simulink model "DriveSystemControl"  (R2025b)
settings: Solver=FixedStepAuto  StartTime=0.0  StopTime=Inf  FixedStep=0.001  RelTol=1e-3
PostLoadFcn:
  | if any(exist('dsrtsu_mdlpostloadfcn', 'file') ~= 0), dsrtsu_mdlpostloadfcn('Execute', bdroot); end
InitFcn:
  | , if any(exist('rtifpga_mdlclblib', 'file') ~= 0), rtifpga_mdlclblib('Init', bdroot); end,
  | , if any(exist('dsmpb_private', 'file') ~= 0), dsmpb_private('dsmpb_mdlclblib', 'Init', bdroot); end,
libraries: dsmpblib x2
(part 2 of 11)

== system DriveSystemControl/Bus Configuration (1) - In/Simulated ECUs/gitam Controller CAN File 08082024/BMS/TX/PDUs/BMS02 ==
  _BMS02_ : BusCreator  Inputs=4
  sigBatteryCurrent : Subsystem
  sigDriveCurrentLimit : Subsystem
  sigRegenCurrentLimit : Subsystem
  sigVehicleModeRequest : Subsystem
  BMS02 : Outport
  wires:
  _BMS02_/1 -> BMS02/1  "BMS02"
  sigVehicleModeRequest/1(sigVehicleModeRequest) -> _BMS02_/1  "sigVehicleModeRequest"
  sigRegenCurrentLimit/1(sigRegenCurrentLimit) -> _BMS02_/2  "sigRegenCurrentLimit"
  sigDriveCurrentLimit/1(sigDriveCurrentLimit) -> _BMS02_/3  "sigDriveCurrentLimit"
  sigBatteryCurrent/1(sigBatteryCurrent) -> _BMS02_/4  "sigBatteryCurrent"

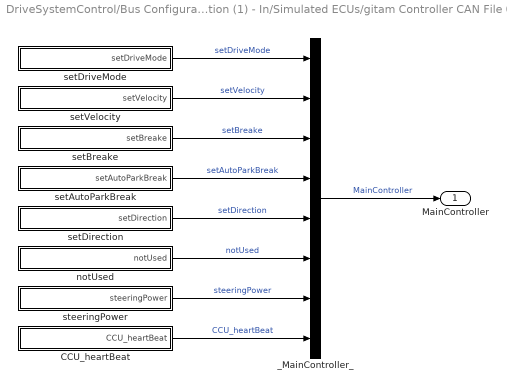
== system DriveSystemControl/Bus Configuration (1) - In/Simulated ECUs/gitam Controller CAN File 08082024/TCU/TX/PDUs/MainController ==
  CCU_heartBeat : Subsystem
  _MainController_ : BusCreator  Inputs=8
  notUsed : Subsystem
  setAutoParkBreak : Subsystem
  setBreake : Subsystem
  setDirection : Subsystem
  setDriveMode : Subsystem
  setVelocity : Subsystem
  steeringPower : Subsystem
  MainController : Outport
  wires:
  _MainController_/1 -> MainController/1  "MainController"
  setDriveMode/1(setDriveMode) -> _MainController_/1  "setDriveMode"
  setVelocity/1(setVelocity) -> _MainController_/2  "setVelocity"
  setBreake/1(setBreake) -> _MainController_/3  "setBreake"
  setAutoParkBreak/1(setAutoParkBreak) -> _MainController_/4  "setAutoParkBreak"
  setDirection/1(setDirection) -> _MainController_/5  "setDirection"
  notUsed/1(notUsed) -> _MainController_/6  "notUsed"
  steeringPower/1(steeringPower) -> _MainController_/7  "steeringPower"
  CCU_heartBeat/1(CCU_heartBeat) -> _MainController_/8  "CCU_heartBeat"

== system DriveSystemControl/Bus Configuration (1) - In/Simulated ECUs/gitam Controller CAN File 08082024/TCU/TX/PDUs/TCU01 ==
  _TCU01_ : BusCreator  Inputs=7
  sigBrake : Subsystem
  sigControllerTemperature : Subsystem
  sigDriveMode : Subsystem
  sigMotorTemperature : Subsystem
  sigRMSCurrent : Subsystem
  sigSpeed : Subsystem
  sigThrottle : Subsystem
  TCU01 : Outport
  wires:
  _TCU01_/1 -> TCU01/1  "TCU01"
  sigBrake/1(sigBrake) -> _TCU01_/1  "sigBrake"
  sigDriveMode/1(sigDriveMode) -> _TCU01_/2  "sigDriveMode"
  sigSpeed/1(sigSpeed) -> _TCU01_/3  "sigSpeed"
  sigThrottle/1(sigThrottle) -> _TCU01_/4  "sigThrottle"
  sigRMSCurrent/1(sigRMSCurrent) -> _TCU01_/5  "sigRMSCurrent"
  sigMotorTemperature/1(sigMotorTemperature) -> _TCU01_/6  "sigMotorTemperature"
  sigControllerTemperature/1(sigControllerTemperature) -> _TCU01_/7  "sigControllerTemperature"

== system DriveSystemControl/Bus Configuration (1) - In/Simulated ECUs/gitam Controller CAN File 08082024/TCU/TX/PDUs/TCU02 ==
  _TCU02_ : BusCreator  Inputs=3
  sigCapacitorVoltage : Subsystem
  sigMotorRPM : Subsystem
  sigOdometer : Subsystem
  TCU02 : Outport
  wires:
  _TCU02_/1 -> TCU02/1  "TCU02"
  sigOdometer/1(sigOdometer) -> _TCU02_/1  "sigOdometer"
  sigCapacitorVoltage/1(sigCapacitorVoltage) -> _TCU02_/2  "sigCapacitorVoltage"
  sigMotorRPM/1(sigMotorRPM) -> _TCU02_/3  "sigMotorRPM"

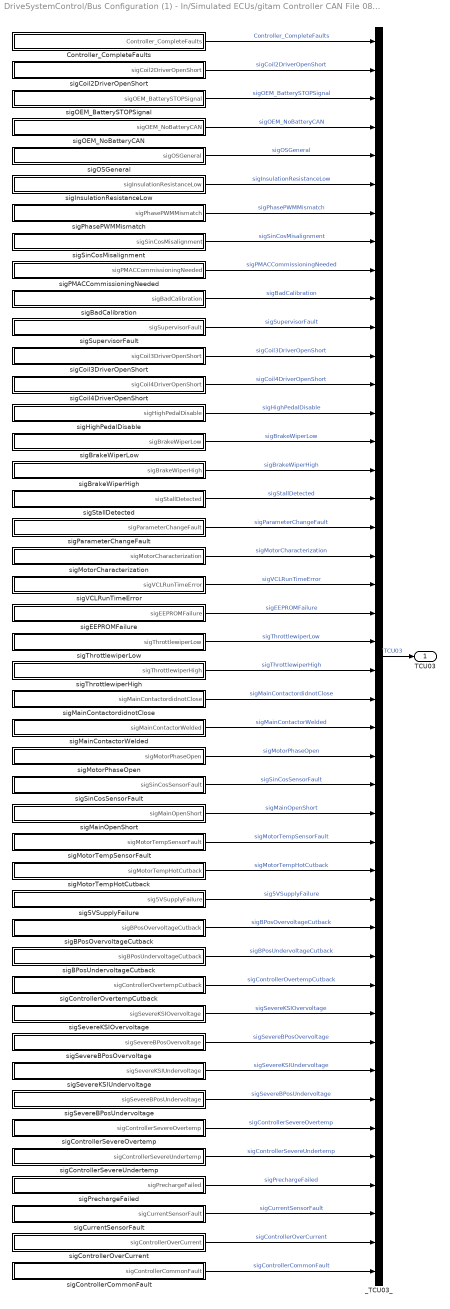
== system DriveSystemControl/Bus Configuration (1) - In/Simulated ECUs/gitam Controller CAN File 08082024/TCU/TX/PDUs/TCU03 ==
  Controller_CompleteFaults : Subsystem
  _TCU03_ : BusCreator  Inputs=44
  sig5VSupplyFailure : Subsystem
  sigBPosOvervoltageCutback : Subsystem
  sigBPosUndervoltageCutback : Subsystem
  sigBadCalibration : Subsystem
  sigBrakeWiperHigh : Subsystem
  sigBrakeWiperLow : Subsystem
  sigCoil2DriverOpenShort : Subsystem
  sigCoil3DriverOpenShort : Subsystem
  sigCoil4DriverOpenShort : Subsystem
  sigControllerCommonFault : Subsystem
  sigControllerOverCurrent : Subsystem
  sigControllerOvertempCutback : Subsystem
  sigControllerSevereOvertemp : Subsystem
  sigControllerSevereUndertemp : Subsystem
  sigCurrentSensorFault : Subsystem
  sigEEPROMFailure : Subsystem
  sigHighPedalDisable : Subsystem
  sigInsulationResistanceLow : Subsystem
  sigMainContactorWelded : Subsystem
  sigMainContactordidnotClose : Subsystem
  sigMainOpenShort : Subsystem
  sigMotorCharacterization : Subsystem
  sigMotorPhaseOpen : Subsystem
  sigMotorTempHotCutback : Subsystem
  sigMotorTempSensorFault : Subsystem
  sigOEM_BatterySTOPSignal : Subsystem
  sigOEM_NoBatteryCAN : Subsystem
  sigOSGeneral : Subsystem
  sigPMACCommissioningNeeded : Subsystem
  sigParameterChangeFault : Subsystem
  sigPhasePWMMismatch : Subsystem
  sigPrechargeFailed : Subsystem
  sigSevereBPosOvervoltage : Subsystem
  sigSevereBPosUndervoltage : Subsystem
  sigSevereKSIOvervoltage : Subsystem
  sigSevereKSIUndervoltage : Subsystem
  sigSinCosMisalignment : Subsystem
  sigSinCosSensorFault : Subsystem
  sigStallDetected : Subsystem
  sigSupervisorFault : Subsystem
  sigThrottlewiperHigh : Subsystem
  sigThrottlewiperLow : Subsystem
  sigVCLRunTimeError : Subsystem
  TCU03 : Outport
  wires:
  _TCU03_/1 -> TCU03/1  "TCU03"
  Controller_CompleteFaults/1(Controller_CompleteFaults) -> _TCU03_/1  "Controller_CompleteFaults"
  sigCoil2DriverOpenShort/1(sigCoil2DriverOpenShort) -> _TCU03_/2  "sigCoil2DriverOpenShort"
  sigOEM_BatterySTOPSignal/1(sigOEM_BatterySTOPSignal) -> _TCU03_/3  "sigOEM_BatterySTOPSignal"
  sigOEM_NoBatteryCAN/1(sigOEM_NoBatteryCAN) -> _TCU03_/4  "sigOEM_NoBatteryCAN"
  sigOSGeneral/1(sigOSGeneral) -> _TCU03_/5  "sigOSGeneral"
  sigInsulationResistanceLow/1(sigInsulationResistanceLow) -> _TCU03_/6  "sigInsulationResistanceLow"
  sigPhasePWMMismatch/1(sigPhasePWMMismatch) -> _TCU03_/7  "sigPhasePWMMismatch"
  sigSinCosMisalignment/1(sigSinCosMisalignment) -> _TCU03_/8  "sigSinCosMisalignment"
  sigPMACCommissioningNeeded/1(sigPMACCommissioningNeeded) -> _TCU03_/9  "sigPMACCommissioningNeeded"
  sigBadCalibration/1(sigBadCalibration) -> _TCU03_/10  "sigBadCalibration"
  sigSupervisorFault/1(sigSupervisorFault) -> _TCU03_/11  "sigSupervisorFault"
  sigCoil3DriverOpenShort/1(sigCoil3DriverOpenShort) -> _TCU03_/12  "sigCoil3DriverOpenShort"
  sigCoil4DriverOpenShort/1(sigCoil4DriverOpenShort) -> _TCU03_/13  "sigCoil4DriverOpenShort"
  sigHighPedalDisable/1(sigHighPedalDisable) -> _TCU03_/14  "sigHighPedalDisable"
  sigBrakeWiperLow/1(sigBrakeWiperLow) -> _TCU03_/15  "sigBrakeWiperLow"
  sigBrakeWiperHigh/1(sigBrakeWiperHigh) -> _TCU03_/16  "sigBrakeWiperHigh"
  sigStallDetected/1(sigStallDetected) -> _TCU03_/17  "sigStallDetected"
  sigParameterChangeFault/1(sigParameterChangeFault) -> _TCU03_/18  "sigParameterChangeFault"
  sigMotorCharacterization/1(sigMotorCharacterization) -> _TCU03_/19  "sigMotorCharacterization"
  sigVCLRunTimeError/1(sigVCLRunTimeError) -> _TCU03_/20  "sigVCLRunTimeError"
  sigEEPROMFailure/1(sigEEPROMFailure) -> _TCU03_/21  "sigEEPROMFailure"
  sigThrottlewiperLow/1(sigThrottlewiperLow) -> _TCU03_/22  "sigThrottlewiperLow"
  sigThrottlewiperHigh/1(sigThrottlewiperHigh) -> _TCU03_/23  "sigThrottlewiperHigh"
  sigMainContactordidnotClose/1(sigMainContactordidnotClose) -> _TCU03_/24  "sigMainContactordidnotClose"
  sigMainContactorWelded/1(sigMainContactorWelded) -> _TCU03_/25  "sigMainContactorWelded"
  sigMotorPhaseOpen/1(sigMotorPhaseOpen) -> _TCU03_/26  "sigMotorPhaseOpen"
  sigSinCosSensorFault/1(sigSinCosSensorFault) -> _TCU03_/27  "sigSinCosSensorFault"
  sigMainOpenShort/1(sigMainOpenShort) -> _TCU03_/28  "sigMainOpenShort"
  sigMotorTempSensorFault/1(sigMotorTempSensorFault) -> _TCU03_/29  "sigMotorTempSensorFault"
  sigMotorTempHotCutback/1(sigMotorTempHotCutback) -> _TCU03_/30  "sigMotorTempHotCutback"
  sig5VSupplyFailure/1(sig5VSupplyFailure) -> _TCU03_/31  "sig5VSupplyFailure"
  sigBPosOvervoltageCutback/1(sigBPosOvervoltageCutback) -> _TCU03_/32  "sigBPosOvervoltageCutback"
  sigBPosUndervoltageCutback/1(sigBPosUndervoltageCutback) -> _TCU03_/33  "sigBPosUndervoltageCutback"
  sigControllerOvertempCutback/1(sigControllerOvertempCutback) -> _TCU03_/34  "sigControllerOvertempCutback"
  sigSevereKSIOvervoltage/1(sigSevereKSIOvervoltage) -> _TCU03_/35  "sigSevereKSIOvervoltage"
  sigSevereBPosOvervoltage/1(sigSevereBPosOvervoltage) -> _TCU03_/36  "sigSevereBPosOvervoltage"
  sigSevereKSIUndervoltage/1(sigSevereKSIUndervoltage) -> _TCU03_/37  "sigSevereKSIUndervoltage"
  sigSevereBPosUndervoltage/1(sigSevereBPosUndervoltage) -> _TCU03_/38  "sigSevereBPosUndervoltage"
  sigControllerSevereOvertemp/1(sigControllerSevereOvertemp) -> _TCU03_/39  "sigControllerSevereOvertemp"
  sigControllerSevereUndertemp/1(sigControllerSevereUndertemp) -> _TCU03_/40  "sigControllerSevereUndertemp"
  sigPrechargeFailed/1(sigPrechargeFailed) -> _TCU03_/41  "sigPrechargeFailed"
  sigCurrentSensorFault/1(sigCurrentSensorFault) -> _TCU03_/42  "sigCurrentSensorFault"
  sigControllerOverCurrent/1(sigControllerOverCurrent) -> _TCU03_/43  "sigControllerOverCurrent"
  sigControllerCommonFault/1(sigControllerCommonFault) -> _TCU03_/44  "sigControllerCommonFault"

== system DriveSystemControl/Bus Configuration (1) - In/Simulated ECUs/gitam Controller CAN File 08082024/TCU/TX/PDUs/TCU04 ==
  _TCU04_ : BusCreator  Inputs=5
  sigMCU5_DriveMode : Subsystem
  sigMCU5_Efficiency : Subsystem
  sigMCU5_Hillhold : Subsystem
  sigMCU5_RegenFlag : Subsystem
  sigMCU5_Speed : Subsystem
  TCU04 : Outport
  wires:
  _TCU04_/1 -> TCU04/1  "TCU04"
  sigMCU5_Efficiency/1(sigMCU5_Efficiency) -> _TCU04_/1  "sigMCU5_Efficiency"
  sigMCU5_Hillhold/1(sigMCU5_Hillhold) -> _TCU04_/2  "sigMCU5_Hillhold"
  sigMCU5_Speed/1(sigMCU5_Speed) -> _TCU04_/3  "sigMCU5_Speed"
  sigMCU5_RegenFlag/1(sigMCU5_RegenFlag) -> _TCU04_/4  "sigMCU5_RegenFlag"
  sigMCU5_DriveMode/1(sigMCU5_DriveMode) -> _TCU04_/5  "sigMCU5_DriveMode"

== system DriveSystemControl/Bus Configuration (1) - In/Simulated ECUs/gitam Controller CAN File 08082024/TCU/TX/PDUs/TCU05 ==
  _TCU05_ : BusCreator  Inputs=1
  sigMCU6_Odometer : Subsystem
  TCU05 : Outport
  wires:
  _TCU05_/1 -> TCU05/1  "TCU05"
  sigMCU6_Odometer/1(sigMCU6_Odometer) -> _TCU05_/1  "sigMCU6_Odometer"

== system DriveSystemControl/Bus Configuration (1) - Out/Manipulation/gitam Controller CAN File 08082024/WIP/CANChannel/PDUs/BMS01 ==
  BMS01 : Inport
  _BMS01_ : BusSelector  OutputSignals=sigBatteryMalfunctionLight,sigKeyOnIndicator,sigStateOfCharge
  sigBatteryMalfunctionLight : Subsystem
  sigKeyOnIndicator : Subsystem
  sigStateOfCharge : Subsystem
  wires:
  BMS01/1 -> _BMS01_/1  "BMS01"
  _BMS01_/1 -> sigBatteryMalfunctionLight/1(sigBatteryMalfunctionLight)  "<sigBatteryMalfunctionLight>"
  _BMS01_/2 -> sigKeyOnIndicator/1(sigKeyOnIndicator)  "<sigKeyOnIndicator>"
  _BMS01_/3 -> sigStateOfCharge/1(sigStateOfCharge)  "<sigStateOfCharge>"

== system DriveSystemControl/Bus Configuration (1) - Out/Manipulation/gitam Controller CAN File 08082024/WIP/CANChannel/PDUs/BMS02 ==
  BMS02 : Inport
  _BMS02_ : BusSelector  OutputSignals=sigVehicleModeRequest,sigRegenCurrentLimit,sigDriveCurrentLimit,sigBatteryCurrent
  sigBatteryCurrent : Subsystem
  sigDriveCurrentLimit : Subsystem
  sigRegenCurrentLimit : Subsystem
  sigVehicleModeRequest : Subsystem
  wires:
  BMS02/1 -> _BMS02_/1  "BMS02"
  _BMS02_/1 -> sigVehicleModeRequest/1(sigVehicleModeRequest)  "<sigVehicleModeRequest>"
  _BMS02_/2 -> sigRegenCurrentLimit/1(sigRegenCurrentLimit)  "<sigRegenCurrentLimit>"
  _BMS02_/3 -> sigDriveCurrentLimit/1(sigDriveCurrentLimit)  "<sigDriveCurrentLimit>"
  _BMS02_/4 -> sigBatteryCurrent/1(sigBatteryCurrent)  "<sigBatteryCurrent>"

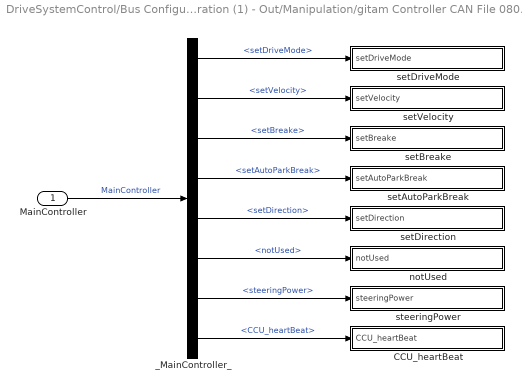
== system DriveSystemControl/Bus Configuration (1) - Out/Manipulation/gitam Controller CAN File 08082024/WIP/CANChannel/PDUs/MainController ==
  MainController : Inport
  CCU_heartBeat : Subsystem
  _MainController_ : BusSelector  OutputSignals=setDriveMode,setVelocity,setBreake,setAutoParkBreak,setDirection,notUsed,steeringPower,CCU_heartBeat
  notUsed : Subsystem
  setAutoParkBreak : Subsystem
  setBreake : Subsystem
  setDirection : Subsystem
  setDriveMode : Subsystem
  setVelocity : Subsystem
  steeringPower : Subsystem
  wires:
  MainController/1 -> _MainController_/1  "MainController"
  _MainController_/1 -> setDriveMode/1(setDriveMode)  "<setDriveMode>"
  _MainController_/2 -> setVelocity/1(setVelocity)  "<setVelocity>"
  _MainController_/3 -> setBreake/1(setBreake)  "<setBreake>"
  _MainController_/4 -> setAutoParkBreak/1(setAutoParkBreak)  "<setAutoParkBreak>"
  _MainController_/5 -> setDirection/1(setDirection)  "<setDirection>"
  _MainController_/6 -> notUsed/1(notUsed)  "<notUsed>"
  _MainController_/7 -> steeringPower/1(steeringPower)  "<steeringPower>"
  _MainController_/8 -> CCU_heartBeat/1(CCU_heartBeat)  "<CCU_heartBeat>"

== system DriveSystemControl/Bus Configuration (1) - Out/Manipulation/gitam Controller CAN File 08082024/WIP/CANChannel/PDUs/TCU01 ==
  TCU01 : Inport
  _TCU01_ : BusSelector  OutputSignals=sigBrake,sigDriveMode,sigSpeed,sigThrottle,sigRMSCurrent,sigMotorTemperature,sigControllerTemperature
  sigBrake : Subsystem
  sigControllerTemperature : Subsystem
  sigDriveMode : Subsystem
  sigMotorTemperature : Subsystem
  sigRMSCurrent : Subsystem
  sigSpeed : Subsystem
  sigThrottle : Subsystem
  wires:
  TCU01/1 -> _TCU01_/1  "TCU01"
  _TCU01_/1 -> sigBrake/1(sigBrake)  "<sigBrake>"
  _TCU01_/2 -> sigDriveMode/1(sigDriveMode)  "<sigDriveMode>"
  _TCU01_/3 -> sigSpeed/1(sigSpeed)  "<sigSpeed>"
  _TCU01_/4 -> sigThrottle/1(sigThrottle)  "<sigThrottle>"
  _TCU01_/5 -> sigRMSCurrent/1(sigRMSCurrent)  "<sigRMSCurrent>"
  _TCU01_/6 -> sigMotorTemperature/1(sigMotorTemperature)  "<sigMotorTemperature>"
  _TCU01_/7 -> sigControllerTemperature/1(sigControllerTemperature)  "<sigControllerTemperature>"

== system DriveSystemControl/Bus Configuration (1) - Out/Manipulation/gitam Controller CAN File 08082024/WIP/CANChannel/PDUs/TCU02 ==
  TCU02 : Inport
  _TCU02_ : BusSelector  OutputSignals=sigOdometer,sigCapacitorVoltage,sigMotorRPM
  sigCapacitorVoltage : Subsystem
  sigMotorRPM : Subsystem
  sigOdometer : Subsystem
  wires:
  TCU02/1 -> _TCU02_/1  "TCU02"
  _TCU02_/1 -> sigOdometer/1(sigOdometer)  "<sigOdometer>"
  _TCU02_/2 -> sigCapacitorVoltage/1(sigCapacitorVoltage)  "<sigCapacitorVoltage>"
  _TCU02_/3 -> sigMotorRPM/1(sigMotorRPM)  "<sigMotorRPM>"

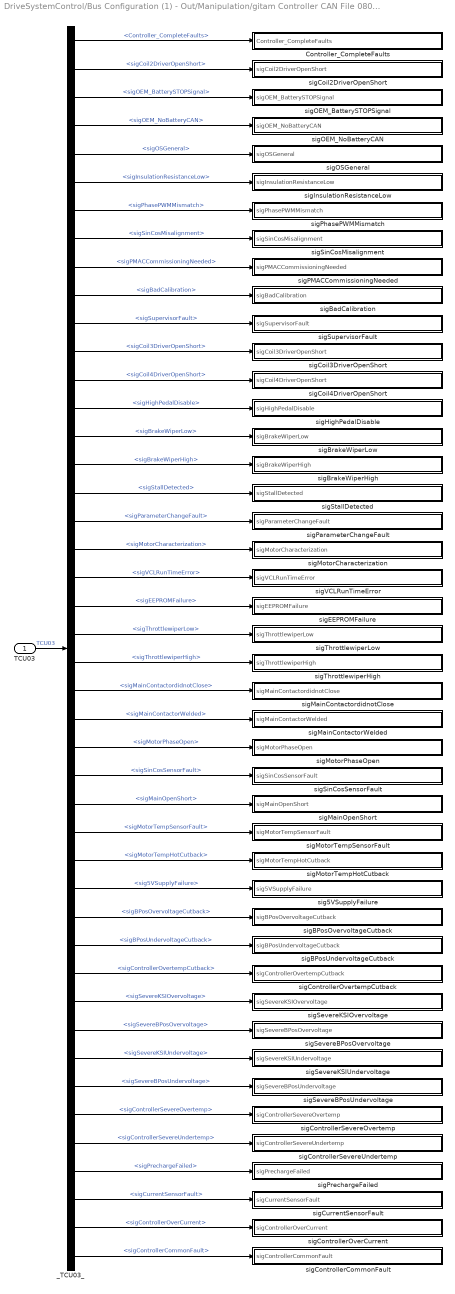
== system DriveSystemControl/Bus Configuration (1) - Out/Manipulation/gitam Controller CAN File 08082024/WIP/CANChannel/PDUs/TCU03 ==
  TCU03 : Inport
  Controller_CompleteFaults : Subsystem
  _TCU03_ : BusSelector  OutputSignals=Controller_CompleteFaults,sigCoil2DriverOpenShort,sigOEM_BatterySTOPSignal,sigOEM_NoBatteryCAN,sigOSGeneral,sigInsulationResistanceLow,sigPhasePWMMismatch,sigSinCosMisalignment,sigPMACCommissioningNeeded,sigBadCalibration,sigSupervisorFault,sigCoil3DriverOpenShort,sigCoil4DriverOpenShort,sigHighPedalDisable,sigBrakeWiperLow,sigBrakeWiperHigh,sigStallDetected,sigParameterChangeFault,sigMotorCharacterization,sigVCLRunTimeError,sigEEPROMFailure,sigThrottlewiperLow,sigThrottlewiperHigh,sigMainContactordidnotClose,sigMainContactorWelded,sigMotorPhaseOpen,sigSinCosSensorFault,sigMainOpenShort,sigMotorTempSensorFault,sigMotorTempHotCutback,sig5VSupplyFailure,sigBPosOvervoltageCutback,sigBPosUndervoltageCutback,sigControllerOvertempCutback,sigSevereKSIOvervoltage,sigSevereBPosOvervoltage,sigSevereKSIUndervoltage,sigSevereBPosUndervoltage,sigControllerSevereOvertemp,sigControllerSevereUndertemp,sigPrechargeFailed,sigCurrentSensorFault,sigControllerOverCurrent,sigControllerCommonFault
  sig5VSupplyFailure : Subsystem
  sigBPosOvervoltageCutback : Subsystem
  sigBPosUndervoltageCutback : Subsystem
  sigBadCalibration : Subsystem
  sigBrakeWiperHigh : Subsystem
  sigBrakeWiperLow : Subsystem
  sigCoil2DriverOpenShort : Subsystem
  sigCoil3DriverOpenShort : Subsystem
  sigCoil4DriverOpenShort : Subsystem
  sigControllerCommonFault : Subsystem
  sigControllerOverCurrent : Subsystem
  sigControllerOvertempCutback : Subsystem
  sigControllerSevereOvertemp : Subsystem
  sigControllerSevereUndertemp : Subsystem
  sigCurrentSensorFault : Subsystem
  sigEEPROMFailure : Subsystem
  sigHighPedalDisable : Subsystem
  sigInsulationResistanceLow : Subsystem
  sigMainContactorWelded : Subsystem
  sigMainContactordidnotClose : Subsystem
  sigMainOpenShort : Subsystem
  sigMotorCharacterization : Subsystem
  sigMotorPhaseOpen : Subsystem
  sigMotorTempHotCutback : Subsystem
  sigMotorTempSensorFault : Subsystem
  sigOEM_BatterySTOPSignal : Subsystem
  sigOEM_NoBatteryCAN : Subsystem
  sigOSGeneral : Subsystem
  sigPMACCommissioningNeeded : Subsystem
  sigParameterChangeFault : Subsystem
  sigPhasePWMMismatch : Subsystem
  sigPrechargeFailed : Subsystem
  sigSevereBPosOvervoltage : Subsystem
  sigSevereBPosUndervoltage : Subsystem
  sigSevereKSIOvervoltage : Subsystem
  sigSevereKSIUndervoltage : Subsystem
  sigSinCosMisalignment : Subsystem
  sigSinCosSensorFault : Subsystem
  sigStallDetected : Subsystem
  sigSupervisorFault : Subsystem
  sigThrottlewiperHigh : Subsystem
  sigThrottlewiperLow : Subsystem
  sigVCLRunTimeError : Subsystem
  wires:
  TCU03/1 -> _TCU03_/1  "TCU03"
  _TCU03_/1 -> Controller_CompleteFaults/1(Controller_CompleteFaults)  "<Controller_CompleteFaults>"
  _TCU03_/2 -> sigCoil2DriverOpenShort/1(sigCoil2DriverOpenShort)  "<sigCoil2DriverOpenShort>"
  _TCU03_/3 -> sigOEM_BatterySTOPSignal/1(sigOEM_BatterySTOPSignal)  "<sigOEM_BatterySTOPSignal>"
  _TCU03_/4 -> sigOEM_NoBatteryCAN/1(sigOEM_NoBatteryCAN)  "<sigOEM_NoBatteryCAN>"
  _TCU03_/5 -> sigOSGeneral/1(sigOSGeneral)  "<sigOSGeneral>"
  _TCU03_/6 -> sigInsulationResistanceLow/1(sigInsulationResistanceLow)  "<sigInsulationResistanceLow>"
  _TCU03_/7 -> sigPhasePWMMismatch/1(sigPhasePWMMismatch)  "<sigPhasePWMMismatch>"
  _TCU03_/8 -> sigSinCosMisalignment/1(sigSinCosMisalignment)  "<sigSinCosMisalignment>"
  _TCU03_/9 -> sigPMACCommissioningNeeded/1(sigPMACCommissioningNeeded)  "<sigPMACCommissioningNeeded>"
  _TCU03_/10 -> sigBadCalibration/1(sigBadCalibration)  "<sigBadCalibration>"
  _TCU03_/11 -> sigSupervisorFault/1(sigSupervisorFault)  "<sigSupervisorFault>"
  _TCU03_/12 -> sigCoil3DriverOpenShort/1(sigCoil3DriverOpenShort)  "<sigCoil3DriverOpenShort>"
  _TCU03_/13 -> sigCoil4DriverOpenShort/1(sigCoil4DriverOpenShort)  "<sigCoil4DriverOpenShort>"
  _TCU03_/14 -> sigHighPedalDisable/1(sigHighPedalDisable)  "<sigHighPedalDisable>"
  _TCU03_/15 -> sigBrakeWiperLow/1(sigBrakeWiperLow)  "<sigBrakeWiperLow>"
  _TCU03_/16 -> sigBrakeWiperHigh/1(sigBrakeWiperHigh)  "<sigBrakeWiperHigh>"
  _TCU03_/17 -> sigStallDetected/1(sigStallDetected)  "<sigStallDetected>"
  _TCU03_/18 -> sigParameterChangeFault/1(sigParameterChangeFault)  "<sigParameterChangeFault>"
  _TCU03_/19 -> sigMotorCharacterization/1(sigMotorCharacterization)  "<sigMotorCharacterization>"
  _TCU03_/20 -> sigVCLRunTimeError/1(sigVCLRunTimeError)  "<sigVCLRunTimeError>"
  _TCU03_/21 -> sigEEPROMFailure/1(sigEEPROMFailure)  "<sigEEPROMFailure>"
  _TCU03_/22 -> sigThrottlewiperLow/1(sigThrottlewiperLow)  "<sigThrottlewiperLow>"
  _TCU03_/23 -> sigThrottlewiperHigh/1(sigThrottlewiperHigh)  "<sigThrottlewiperHigh>"
  _TCU03_/24 -> sigMainContactordidnotClose/1(sigMainContactordidnotClose)  "<sigMainContactordidnotClose>"
  _TCU03_/25 -> sigMainContactorWelded/1(sigMainContactorWelded)  "<sigMainContactorWelded>"
  _TCU03_/26 -> sigMotorPhaseOpen/1(sigMotorPhaseOpen)  "<sigMotorPhaseOpen>"
  _TCU03_/27 -> sigSinCosSensorFault/1(sigSinCosSensorFault)  "<sigSinCosSensorFault>"
  _TCU03_/28 -> sigMainOpenShort/1(sigMainOpenShort)  "<sigMainOpenShort>"
  _TCU03_/29 -> sigMotorTempSensorFault/1(sigMotorTempSensorFault)  "<sigMotorTempSensorFault>"
  _TCU03_/30 -> sigMotorTempHotCutback/1(sigMotorTempHotCutback)  "<sigMotorTempHotCutback>"
  _TCU03_/31 -> sig5VSupplyFailure/1(sig5VSupplyFailure)  "<sig5VSupplyFailure>"
  _TCU03_/32 -> sigBPosOvervoltageCutback/1(sigBPosOvervoltageCutback)  "<sigBPosOvervoltageCutback>"
  _TCU03_/33 -> sigBPosUndervoltageCutback/1(sigBPosUndervoltageCutback)  "<sigBPosUndervoltageCutback>"
  _TCU03_/34 -> sigControllerOvertempCutback/1(sigControllerOvertempCutback)  "<sigControllerOvertempCutback>"
  _TCU03_/35 -> sigSevereKSIOvervoltage/1(sigSevereKSIOvervoltage)  "<sigSevereKSIOvervoltage>"
  _TCU03_/36 -> sigSevereBPosOvervoltage/1(sigSevereBPosOvervoltage)  "<sigSevereBPosOvervoltage>"
  _TCU03_/37 -> sigSevereKSIUndervoltage/1(sigSevereKSIUndervoltage)  "<sigSevereKSIUndervoltage>"
  _TCU03_/38 -> sigSevereBPosUndervoltage/1(sigSevereBPosUndervoltage)  "<sigSevereBPosUndervoltage>"
  _TCU03_/39 -> sigControllerSevereOvertemp/1(sigControllerSevereOvertemp)  "<sigControllerSevereOvertemp>"
  _TCU03_/40 -> sigControllerSevereUndertemp/1(sigControllerSevereUndertemp)  "<sigControllerSevereUndertemp>"
  _TCU03_/41 -> sigPrechargeFailed/1(sigPrechargeFailed)  "<sigPrechargeFailed>"
  _TCU03_/42 -> sigCurrentSensorFault/1(sigCurrentSensorFault)  "<sigCurrentSensorFault>"
  _TCU03_/43 -> sigControllerOverCurrent/1(sigControllerOverCurrent)  "<sigControllerOverCurrent>"
  _TCU03_/44 -> sigControllerCommonFault/1(sigControllerCommonFault)  "<sigControllerCommonFault>"

== system DriveSystemControl/Bus Configuration (1) - Out/Manipulation/gitam Controller CAN File 08082024/WIP/CANChannel/PDUs/TCU04 ==
  TCU04 : Inport
  _TCU04_ : BusSelector  OutputSignals=sigMCU5_Efficiency,sigMCU5_Hillhold,sigMCU5_Speed,sigMCU5_RegenFlag,sigMCU5_DriveMode
  sigMCU5_DriveMode : Subsystem
  sigMCU5_Efficiency : Subsystem
  sigMCU5_Hillhold : Subsystem
  sigMCU5_RegenFlag : Subsystem
  sigMCU5_Speed : Subsystem
  wires:
  TCU04/1 -> _TCU04_/1  "TCU04"
  _TCU04_/1 -> sigMCU5_Efficiency/1(sigMCU5_Efficiency)  "<sigMCU5_Efficiency>"
  _TCU04_/2 -> sigMCU5_Hillhold/1(sigMCU5_Hillhold)  "<sigMCU5_Hillhold>"
  _TCU04_/3 -> sigMCU5_Speed/1(sigMCU5_Speed)  "<sigMCU5_Speed>"
  _TCU04_/4 -> sigMCU5_RegenFlag/1(sigMCU5_RegenFlag)  "<sigMCU5_RegenFlag>"
  _TCU04_/5 -> sigMCU5_DriveMode/1(sigMCU5_DriveMode)  "<sigMCU5_DriveMode>"

== system DriveSystemControl/Bus Configuration (1) - Out/Manipulation/gitam Controller CAN File 08082024/WIP/CANChannel/PDUs/TCU05 ==
  TCU05 : Inport
  _TCU05_ : BusSelector  OutputSignals=sigMCU6_Odometer
  sigMCU6_Odometer : Subsystem
  wires:
  TCU05/1 -> _TCU05_/1  "TCU05"
  _TCU05_/1 -> sigMCU6_Odometer/1(sigMCU6_Odometer)  "<sigMCU6_Odometer>"

== system DriveSystemControl/Bus Configuration (1) - Out/Simulated ECUs/gitam Controller CAN File 08082024/BMS/RX/PDUs/TCU04 ==
  TCU04 : Inport
  _TCU04_ : BusSelector  OutputSignals=sigMCU5_Efficiency,sigMCU5_Hillhold,sigMCU5_Speed,sigMCU5_RegenFlag,sigMCU5_DriveMode
  sigMCU5_DriveMode : Subsystem
  sigMCU5_Efficiency : Subsystem
  sigMCU5_Hillhold : Subsystem
  sigMCU5_RegenFlag : Subsystem
  sigMCU5_Speed : Subsystem
  wires:
  TCU04/1 -> _TCU04_/1  "TCU04"
  _TCU04_/1 -> sigMCU5_Efficiency/1(sigMCU5_Efficiency)  "<sigMCU5_Efficiency>"
  _TCU04_/2 -> sigMCU5_Hillhold/1(sigMCU5_Hillhold)  "<sigMCU5_Hillhold>"
  _TCU04_/3 -> sigMCU5_Speed/1(sigMCU5_Speed)  "<sigMCU5_Speed>"
  _TCU04_/4 -> sigMCU5_RegenFlag/1(sigMCU5_RegenFlag)  "<sigMCU5_RegenFlag>"
  _TCU04_/5 -> sigMCU5_DriveMode/1(sigMCU5_DriveMode)  "<sigMCU5_DriveMode>"

== system DriveSystemControl/Bus Configuration (1) - Out/Simulated ECUs/gitam Controller CAN File 08082024/IPC/RX/PDUs/BMS01 ==
  BMS01 : Inport
  _BMS01_ : BusSelector  OutputSignals=sigBatteryMalfunctionLight,sigKeyOnIndicator,sigStateOfCharge
  sigBatteryMalfunctionLight : Subsystem
  sigKeyOnIndicator : Subsystem
  sigStateOfCharge : Subsystem
  wires:
  BMS01/1 -> _BMS01_/1  "BMS01"
  _BMS01_/1 -> sigBatteryMalfunctionLight/1(sigBatteryMalfunctionLight)  "<sigBatteryMalfunctionLight>"
  _BMS01_/2 -> sigKeyOnIndicator/1(sigKeyOnIndicator)  "<sigKeyOnIndicator>"
  _BMS01_/3 -> sigStateOfCharge/1(sigStateOfCharge)  "<sigStateOfCharge>"

== system DriveSystemControl/Bus Configuration (1) - Out/Simulated ECUs/gitam Controller CAN File 08082024/IPC/RX/PDUs/TCU01 ==
  TCU01 : Inport
  _TCU01_ : BusSelector  OutputSignals=sigBrake,sigDriveMode,sigSpeed,sigThrottle,sigRMSCurrent,sigMotorTemperature,sigControllerTemperature
  sigBrake : Subsystem
  sigControllerTemperature : Subsystem
  sigDriveMode : Subsystem
  sigMotorTemperature : Subsystem
  sigRMSCurrent : Subsystem
  sigSpeed : Subsystem
  sigThrottle : Subsystem
  wires:
  TCU01/1 -> _TCU01_/1  "TCU01"
  _TCU01_/1 -> sigBrake/1(sigBrake)  "<sigBrake>"
  _TCU01_/2 -> sigDriveMode/1(sigDriveMode)  "<sigDriveMode>"
  _TCU01_/3 -> sigSpeed/1(sigSpeed)  "<sigSpeed>"
  _TCU01_/4 -> sigThrottle/1(sigThrottle)  "<sigThrottle>"
  _TCU01_/5 -> sigRMSCurrent/1(sigRMSCurrent)  "<sigRMSCurrent>"
  _TCU01_/6 -> sigMotorTemperature/1(sigMotorTemperature)  "<sigMotorTemperature>"
  _TCU01_/7 -> sigControllerTemperature/1(sigControllerTemperature)  "<sigControllerTemperature>"

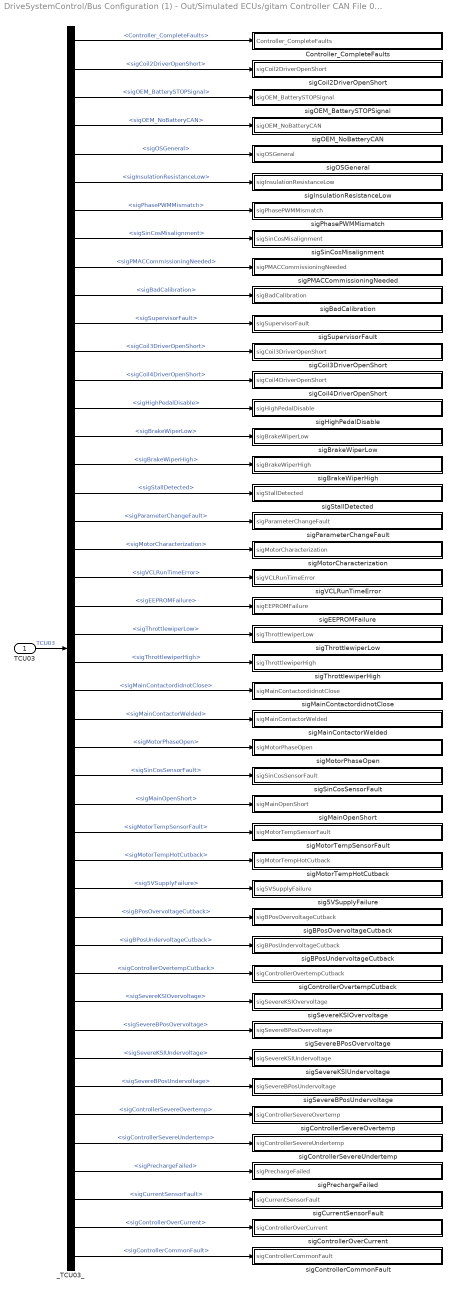
== system DriveSystemControl/Bus Configuration (1) - Out/Simulated ECUs/gitam Controller CAN File 08082024/IPC/RX/PDUs/TCU03 ==
  TCU03 : Inport
  Controller_CompleteFaults : Subsystem
  _TCU03_ : BusSelector  OutputSignals=Controller_CompleteFaults,sigCoil2DriverOpenShort,sigOEM_BatterySTOPSignal,sigOEM_NoBatteryCAN,sigOSGeneral,sigInsulationResistanceLow,sigPhasePWMMismatch,sigSinCosMisalignment,sigPMACCommissioningNeeded,sigBadCalibration,sigSupervisorFault,sigCoil3DriverOpenShort,sigCoil4DriverOpenShort,sigHighPedalDisable,sigBrakeWiperLow,sigBrakeWiperHigh,sigStallDetected,sigParameterChangeFault,sigMotorCharacterization,sigVCLRunTimeError,sigEEPROMFailure,sigThrottlewiperLow,sigThrottlewiperHigh,sigMainContactordidnotClose,sigMainContactorWelded,sigMotorPhaseOpen,sigSinCosSensorFault,sigMainOpenShort,sigMotorTempSensorFault,sigMotorTempHotCutback,sig5VSupplyFailure,sigBPosOvervoltageCutback,sigBPosUndervoltageCutback,sigControllerOvertempCutback,sigSevereKSIOvervoltage,sigSevereBPosOvervoltage,sigSevereKSIUndervoltage,sigSevereBPosUndervoltage,sigControllerSevereOvertemp,sigControllerSevereUndertemp,sigPrechargeFailed,sigCurrentSensorFault,sigControllerOverCurrent,sigControllerCommonFault
  sig5VSupplyFailure : Subsystem
  sigBPosOvervoltageCutback : Subsystem
  sigBPosUndervoltageCutback : Subsystem
  sigBadCalibration : Subsystem
  sigBrakeWiperHigh : Subsystem
  sigBrakeWiperLow : Subsystem
  sigCoil2DriverOpenShort : Subsystem
  sigCoil3DriverOpenShort : Subsystem
  sigCoil4DriverOpenShort : Subsystem
  sigControllerCommonFault : Subsystem
  sigControllerOverCurrent : Subsystem
  sigControllerOvertempCutback : Subsystem
  sigControllerSevereOvertemp : Subsystem
  sigControllerSevereUndertemp : Subsystem
  sigCurrentSensorFault : Subsystem
  sigEEPROMFailure : Subsystem
  sigHighPedalDisable : Subsystem
  sigInsulationResistanceLow : Subsystem
  sigMainContactorWelded : Subsystem
  sigMainContactordidnotClose : Subsystem
  sigMainOpenShort : Subsystem
  sigMotorCharacterization : Subsystem
  sigMotorPhaseOpen : Subsystem
  sigMotorTempHotCutback : Subsystem
  sigMotorTempSensorFault : Subsystem
  sigOEM_BatterySTOPSignal : Subsystem
  sigOEM_NoBatteryCAN : Subsystem
  sigOSGeneral : Subsystem
  sigPMACCommissioningNeeded : Subsystem
  sigParameterChangeFault : Subsystem
  sigPhasePWMMismatch : Subsystem
  sigPrechargeFailed : Subsystem
  sigSevereBPosOvervoltage : Subsystem
  sigSevereBPosUndervoltage : Subsystem
  sigSevereKSIOvervoltage : Subsystem
  sigSevereKSIUndervoltage : Subsystem
  sigSinCosMisalignment : Subsystem
  sigSinCosSensorFault : Subsystem
  sigStallDetected : Subsystem
  sigSupervisorFault : Subsystem
  sigThrottlewiperHigh : Subsystem
  sigThrottlewiperLow : Subsystem
  sigVCLRunTimeError : Subsystem
  wires:
  TCU03/1 -> _TCU03_/1  "TCU03"
  _TCU03_/1 -> Controller_CompleteFaults/1(Controller_CompleteFaults)  "<Controller_CompleteFaults>"
  _TCU03_/2 -> sigCoil2DriverOpenShort/1(sigCoil2DriverOpenShort)  "<sigCoil2DriverOpenShort>"
  _TCU03_/3 -> sigOEM_BatterySTOPSignal/1(sigOEM_BatterySTOPSignal)  "<sigOEM_BatterySTOPSignal>"
  _TCU03_/4 -> sigOEM_NoBatteryCAN/1(sigOEM_NoBatteryCAN)  "<sigOEM_NoBatteryCAN>"
  _TCU03_/5 -> sigOSGeneral/1(sigOSGeneral)  "<sigOSGeneral>"
  _TCU03_/6 -> sigInsulationResistanceLow/1(sigInsulationResistanceLow)  "<sigInsulationResistanceLow>"
  _TCU03_/7 -> sigPhasePWMMismatch/1(sigPhasePWMMismatch)  "<sigPhasePWMMismatch>"
  _TCU03_/8 -> sigSinCosMisalignment/1(sigSinCosMisalignment)  "<sigSinCosMisalignment>"
  _TCU03_/9 -> sigPMACCommissioningNeeded/1(sigPMACCommissioningNeeded)  "<sigPMACCommissioningNeeded>"
  _TCU03_/10 -> sigBadCalibration/1(sigBadCalibration)  "<sigBadCalibration>"
  _TCU03_/11 -> sigSupervisorFault/1(sigSupervisorFault)  "<sigSupervisorFault>"
  _TCU03_/12 -> sigCoil3DriverOpenShort/1(sigCoil3DriverOpenShort)  "<sigCoil3DriverOpenShort>"
  _TCU03_/13 -> sigCoil4DriverOpenShort/1(sigCoil4DriverOpenShort)  "<sigCoil4DriverOpenShort>"
  _TCU03_/14 -> sigHighPedalDisable/1(sigHighPedalDisable)  "<sigHighPedalDisable>"
  _TCU03_/15 -> sigBrakeWiperLow/1(sigBrakeWiperLow)  "<sigBrakeWiperLow>"
  _TCU03_/16 -> sigBrakeWiperHigh/1(sigBrakeWiperHigh)  "<sigBrakeWiperHigh>"
  _TCU03_/17 -> sigStallDetected/1(sigStallDetected)  "<sigStallDetected>"
  _TCU03_/18 -> sigParameterChangeFault/1(sigParameterChangeFault)  "<sigParameterChangeFault>"
  _TCU03_/19 -> sigMotorCharacterization/1(sigMotorCharacterization)  "<sigMotorCharacterization>"
  _TCU03_/20 -> sigVCLRunTimeError/1(sigVCLRunTimeError)  "<sigVCLRunTimeError>"
  _TCU03_/21 -> sigEEPROMFailure/1(sigEEPROMFailure)  "<sigEEPROMFailure>"
  _TCU03_/22 -> sigThrottlewiperLow/1(sigThrottlewiperLow)  "<sigThrottlewiperLow>"
  _TCU03_/23 -> sigThrottlewiperHigh/1(sigThrottlewiperHigh)  "<sigThrottlewiperHigh>"
  _TCU03_/24 -> sigMainContactordidnotClose/1(sigMainContactordidnotClose)  "<sigMainContactordidnotClose>"
  _TCU03_/25 -> sigMainContactorWelded/1(sigMainContactorWelded)  "<sigMainContactorWelded>"
  _TCU03_/26 -> sigMotorPhaseOpen/1(sigMotorPhaseOpen)  "<sigMotorPhaseOpen>"
  _TCU03_/27 -> sigSinCosSensorFault/1(sigSinCosSensorFault)  "<sigSinCosSensorFault>"
  _TCU03_/28 -> sigMainOpenShort/1(sigMainOpenShort)  "<sigMainOpenShort>"
  _TCU03_/29 -> sigMotorTempSensorFault/1(sigMotorTempSensorFault)  "<sigMotorTempSensorFault>"
  _TCU03_/30 -> sigMotorTempHotCutback/1(sigMotorTempHotCutback)  "<sigMotorTempHotCutback>"
  _TCU03_/31 -> sig5VSupplyFailure/1(sig5VSupplyFailure)  "<sig5VSupplyFailure>"
  _TCU03_/32 -> sigBPosOvervoltageCutback/1(sigBPosOvervoltageCutback)  "<sigBPosOvervoltageCutback>"
  _TCU03_/33 -> sigBPosUndervoltageCutback/1(sigBPosUndervoltageCutback)  "<sigBPosUndervoltageCutback>"
  _TCU03_/34 -> sigControllerOvertempCutback/1(sigControllerOvertempCutback)  "<sigControllerOvertempCutback>"
  _TCU03_/35 -> sigSevereKSIOvervoltage/1(sigSevereKSIOvervoltage)  "<sigSevereKSIOvervoltage>"
  _TCU03_/36 -> sigSevereBPosOvervoltage/1(sigSevereBPosOvervoltage)  "<sigSevereBPosOvervoltage>"
  _TCU03_/37 -> sigSevereKSIUndervoltage/1(sigSevereKSIUndervoltage)  "<sigSevereKSIUndervoltage>"
  _TCU03_/38 -> sigSevereBPosUndervoltage/1(sigSevereBPosUndervoltage)  "<sigSevereBPosUndervoltage>"
  _TCU03_/39 -> sigControllerSevereOvertemp/1(sigControllerSevereOvertemp)  "<sigControllerSevereOvertemp>"
  _TCU03_/40 -> sigControllerSevereUndertemp/1(sigControllerSevereUndertemp)  "<sigControllerSevereUndertemp>"
  _TCU03_/41 -> sigPrechargeFailed/1(sigPrechargeFailed)  "<sigPrechargeFailed>"
  _TCU03_/42 -> sigCurrentSensorFault/1(sigCurrentSensorFault)  "<sigCurrentSensorFault>"
  _TCU03_/43 -> sigControllerOverCurrent/1(sigControllerOverCurrent)  "<sigControllerOverCurrent>"
  _TCU03_/44 -> sigControllerCommonFault/1(sigControllerCommonFault)  "<sigControllerCommonFault>"

== system DriveSystemControl/Bus Configuration (1) - Out/Simulated ECUs/gitam Controller CAN File 08082024/IPC/RX/PDUs/TCU04 ==
  TCU04 : Inport
  _TCU04_ : BusSelector  OutputSignals=sigMCU5_Efficiency,sigMCU5_Hillhold,sigMCU5_Speed,sigMCU5_RegenFlag,sigMCU5_DriveMode
  sigMCU5_DriveMode : Subsystem
  sigMCU5_Efficiency : Subsystem
  sigMCU5_Hillhold : Subsystem
  sigMCU5_RegenFlag : Subsystem
  sigMCU5_Speed : Subsystem
  wires:
  TCU04/1 -> _TCU04_/1  "TCU04"
  _TCU04_/1 -> sigMCU5_Efficiency/1(sigMCU5_Efficiency)  "<sigMCU5_Efficiency>"
  _TCU04_/2 -> sigMCU5_Hillhold/1(sigMCU5_Hillhold)  "<sigMCU5_Hillhold>"
  _TCU04_/3 -> sigMCU5_Speed/1(sigMCU5_Speed)  "<sigMCU5_Speed>"
  _TCU04_/4 -> sigMCU5_RegenFlag/1(sigMCU5_RegenFlag)  "<sigMCU5_RegenFlag>"
  _TCU04_/5 -> sigMCU5_DriveMode/1(sigMCU5_DriveMode)  "<sigMCU5_DriveMode>"

== system DriveSystemControl/Bus Configuration (1) - Out/Simulated ECUs/gitam Controller CAN File 08082024/IPC/RX/PDUs/TCU05 ==
  TCU05 : Inport
  _TCU05_ : BusSelector  OutputSignals=sigMCU6_Odometer
  sigMCU6_Odometer : Subsystem
  wires:
  TCU05/1 -> _TCU05_/1  "TCU05"
  _TCU05_/1 -> sigMCU6_Odometer/1(sigMCU6_Odometer)  "<sigMCU6_Odometer>"

== system DriveSystemControl/Bus Configuration (1) - Out/Simulated ECUs/gitam Controller CAN File 08082024/TCU/RX/PDUs/BMS02 ==
  BMS02 : Inport
  _BMS02_ : BusSelector  OutputSignals=sigVehicleModeRequest,sigRegenCurrentLimit,sigDriveCurrentLimit,sigBatteryCurrent
  sigBatteryCurrent : Subsystem
  sigDriveCurrentLimit : Subsystem
  sigRegenCurrentLimit : Subsystem
  sigVehicleModeRequest : Subsystem
  wires:
  BMS02/1 -> _BMS02_/1  "BMS02"
  _BMS02_/1 -> sigVehicleModeRequest/1(sigVehicleModeRequest)  "<sigVehicleModeRequest>"
  _BMS02_/2 -> sigRegenCurrentLimit/1(sigRegenCurrentLimit)  "<sigRegenCurrentLimit>"
  _BMS02_/3 -> sigDriveCurrentLimit/1(sigDriveCurrentLimit)  "<sigDriveCurrentLimit>"
  _BMS02_/4 -> sigBatteryCurrent/1(sigBatteryCurrent)  "<sigBatteryCurrent>"

== system DriveSystemControl/Bus Configuration (1) - Out/Simulated ECUs/gitam Controller CAN File 08082024/Telematics/RX/PDUs/BMS01 ==
  BMS01 : Inport
  _BMS01_ : BusSelector  OutputSignals=sigBatteryMalfunctionLight,sigKeyOnIndicator,sigStateOfCharge
  sigBatteryMalfunctionLight : Subsystem
  sigKeyOnIndicator : Subsystem
  sigStateOfCharge : Subsystem
  wires:
  BMS01/1 -> _BMS01_/1  "BMS01"
  _BMS01_/1 -> sigBatteryMalfunctionLight/1(sigBatteryMalfunctionLight)  "<sigBatteryMalfunctionLight>"
  _BMS01_/2 -> sigKeyOnIndicator/1(sigKeyOnIndicator)  "<sigKeyOnIndicator>"
  _BMS01_/3 -> sigStateOfCharge/1(sigStateOfCharge)  "<sigStateOfCharge>"

== system DriveSystemControl/Bus Configuration (1) - Out/Simulated ECUs/gitam Controller CAN File 08082024/Telematics/RX/PDUs/BMS02 ==
  BMS02 : Inport
  _BMS02_ : BusSelector  OutputSignals=sigVehicleModeRequest,sigRegenCurrentLimit,sigDriveCurrentLimit,sigBatteryCurrent
  sigBatteryCurrent : Subsystem
  sigDriveCurrentLimit : Subsystem
  sigRegenCurrentLimit : Subsystem
  sigVehicleModeRequest : Subsystem
  wires:
  BMS02/1 -> _BMS02_/1  "BMS02"
  _BMS02_/1 -> sigVehicleModeRequest/1(sigVehicleModeRequest)  "<sigVehicleModeRequest>"
  _BMS02_/2 -> sigRegenCurrentLimit/1(sigRegenCurrentLimit)  "<sigRegenCurrentLimit>"
  _BMS02_/3 -> sigDriveCurrentLimit/1(sigDriveCurrentLimit)  "<sigDriveCurrentLimit>"
  _BMS02_/4 -> sigBatteryCurrent/1(sigBatteryCurrent)  "<sigBatteryCurrent>"

== system DriveSystemControl/Bus Configuration (1) - Out/Simulated ECUs/gitam Controller CAN File 08082024/Telematics/RX/PDUs/TCU01 ==
  TCU01 : Inport
  _TCU01_ : BusSelector  OutputSignals=sigBrake,sigDriveMode,sigSpeed,sigThrottle,sigRMSCurrent,sigMotorTemperature,sigControllerTemperature
  sigBrake : Subsystem
  sigControllerTemperature : Subsystem
  sigDriveMode : Subsystem
  sigMotorTemperature : Subsystem
  sigRMSCurrent : Subsystem
  sigSpeed : Subsystem
  sigThrottle : Subsystem
  wires:
  TCU01/1 -> _TCU01_/1  "TCU01"
  _TCU01_/1 -> sigBrake/1(sigBrake)  "<sigBrake>"
  _TCU01_/2 -> sigDriveMode/1(sigDriveMode)  "<sigDriveMode>"
  _TCU01_/3 -> sigSpeed/1(sigSpeed)  "<sigSpeed>"
  _TCU01_/4 -> sigThrottle/1(sigThrottle)  "<sigThrottle>"
  _TCU01_/5 -> sigRMSCurrent/1(sigRMSCurrent)  "<sigRMSCurrent>"
  _TCU01_/6 -> sigMotorTemperature/1(sigMotorTemperature)  "<sigMotorTemperature>"
  _TCU01_/7 -> sigControllerTemperature/1(sigControllerTemperature)  "<sigControllerTemperature>"

== system DriveSystemControl/Bus Configuration (1) - Out/Simulated ECUs/gitam Controller CAN File 08082024/Telematics/RX/PDUs/TCU02 ==
  TCU02 : Inport
  _TCU02_ : BusSelector  OutputSignals=sigOdometer,sigCapacitorVoltage,sigMotorRPM
  sigCapacitorVoltage : Subsystem
  sigMotorRPM : Subsystem
  sigOdometer : Subsystem
  wires:
  TCU02/1 -> _TCU02_/1  "TCU02"
  _TCU02_/1 -> sigOdometer/1(sigOdometer)  "<sigOdometer>"
  _TCU02_/2 -> sigCapacitorVoltage/1(sigCapacitorVoltage)  "<sigCapacitorVoltage>"
  _TCU02_/3 -> sigMotorRPM/1(sigMotorRPM)  "<sigMotorRPM>"

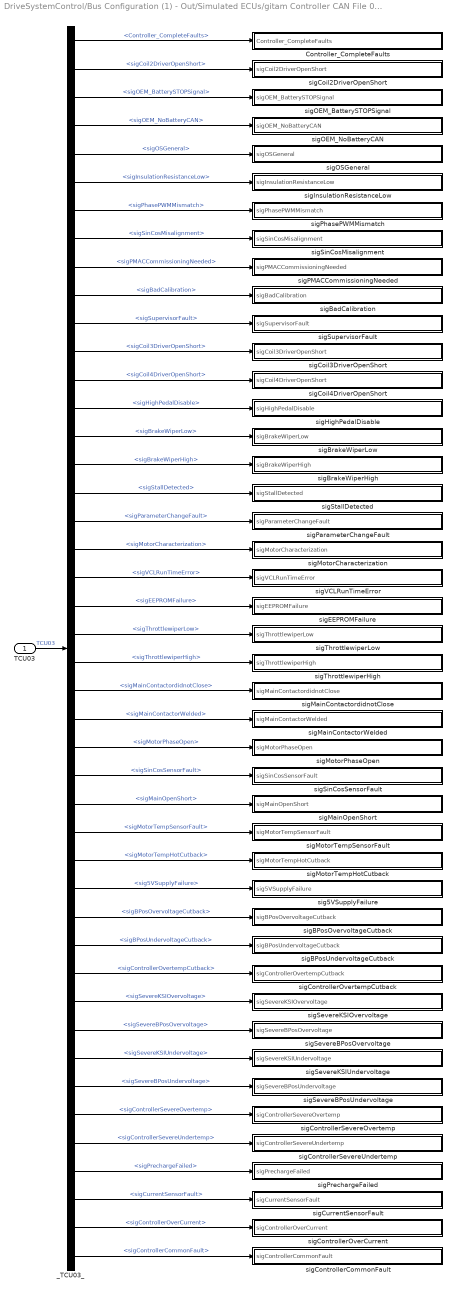
== system DriveSystemControl/Bus Configuration (1) - Out/Simulated ECUs/gitam Controller CAN File 08082024/Telematics/RX/PDUs/TCU03 ==
  TCU03 : Inport
  Controller_CompleteFaults : Subsystem
  _TCU03_ : BusSelector  OutputSignals=Controller_CompleteFaults,sigCoil2DriverOpenShort,sigOEM_BatterySTOPSignal,sigOEM_NoBatteryCAN,sigOSGeneral,sigInsulationResistanceLow,sigPhasePWMMismatch,sigSinCosMisalignment,sigPMACCommissioningNeeded,sigBadCalibration,sigSupervisorFault,sigCoil3DriverOpenShort,sigCoil4DriverOpenShort,sigHighPedalDisable,sigBrakeWiperLow,sigBrakeWiperHigh,sigStallDetected,sigParameterChangeFault,sigMotorCharacterization,sigVCLRunTimeError,sigEEPROMFailure,sigThrottlewiperLow,sigThrottlewiperHigh,sigMainContactordidnotClose,sigMainContactorWelded,sigMotorPhaseOpen,sigSinCosSensorFault,sigMainOpenShort,sigMotorTempSensorFault,sigMotorTempHotCutback,sig5VSupplyFailure,sigBPosOvervoltageCutback,sigBPosUndervoltageCutback,sigControllerOvertempCutback,sigSevereKSIOvervoltage,sigSevereBPosOvervoltage,sigSevereKSIUndervoltage,sigSevereBPosUndervoltage,sigControllerSevereOvertemp,sigControllerSevereUndertemp,sigPrechargeFailed,sigCurrentSensorFault,sigControllerOverCurrent,sigControllerCommonFault
  sig5VSupplyFailure : Subsystem
  sigBPosOvervoltageCutback : Subsystem
  sigBPosUndervoltageCutback : Subsystem
  sigBadCalibration : Subsystem
  sigBrakeWiperHigh : Subsystem
  sigBrakeWiperLow : Subsystem
  sigCoil2DriverOpenShort : Subsystem
  sigCoil3DriverOpenShort : Subsystem
  sigCoil4DriverOpenShort : Subsystem
  sigControllerCommonFault : Subsystem
  sigControllerOverCurrent : Subsystem
  sigControllerOvertempCutback : Subsystem
  sigControllerSevereOvertemp : Subsystem
  sigControllerSevereUndertemp : Subsystem
  sigCurrentSensorFault : Subsystem
  sigEEPROMFailure : Subsystem
  sigHighPedalDisable : Subsystem
  sigInsulationResistanceLow : Subsystem
  sigMainContactorWelded : Subsystem
  sigMainContactordidnotClose : Subsystem
  sigMainOpenShort : Subsystem
  sigMotorCharacterization : Subsystem
  sigMotorPhaseOpen : Subsystem
  sigMotorTempHotCutback : Subsystem
  sigMotorTempSensorFault : Subsystem
  sigOEM_BatterySTOPSignal : Subsystem
  sigOEM_NoBatteryCAN : Subsystem
  sigOSGeneral : Subsystem
  sigPMACCommissioningNeeded : Subsystem
  sigParameterChangeFault : Subsystem
  sigPhasePWMMismatch : Subsystem
  sigPrechargeFailed : Subsystem
  sigSevereBPosOvervoltage : Subsystem
  sigSevereBPosUndervoltage : Subsystem
  sigSevereKSIOvervoltage : Subsystem
  sigSevereKSIUndervoltage : Subsystem
  sigSinCosMisalignment : Subsystem
  sigSinCosSensorFault : Subsystem
  sigStallDetected : Subsystem
  sigSupervisorFault : Subsystem
  sigThrottlewiperHigh : Subsystem
  sigThrottlewiperLow : Subsystem
  sigVCLRunTimeError : Subsystem
  wires:
  TCU03/1 -> _TCU03_/1  "TCU03"
  _TCU03_/1 -> Controller_CompleteFaults/1(Controller_CompleteFaults)  "<Controller_CompleteFaults>"
  _TCU03_/2 -> sigCoil2DriverOpenShort/1(sigCoil2DriverOpenShort)  "<sigCoil2DriverOpenShort>"
  _TCU03_/3 -> sigOEM_BatterySTOPSignal/1(sigOEM_BatterySTOPSignal)  "<sigOEM_BatterySTOPSignal>"
  _TCU03_/4 -> sigOEM_NoBatteryCAN/1(sigOEM_NoBatteryCAN)  "<sigOEM_NoBatteryCAN>"
  _TCU03_/5 -> sigOSGeneral/1(sigOSGeneral)  "<sigOSGeneral>"
  _TCU03_/6 -> sigInsulationResistanceLow/1(sigInsulationResistanceLow)  "<sigInsulationResistanceLow>"
  _TCU03_/7 -> sigPhasePWMMismatch/1(sigPhasePWMMismatch)  "<sigPhasePWMMismatch>"
  _TCU03_/8 -> sigSinCosMisalignment/1(sigSinCosMisalignment)  "<sigSinCosMisalignment>"
  _TCU03_/9 -> sigPMACCommissioningNeeded/1(sigPMACCommissioningNeeded)  "<sigPMACCommissioningNeeded>"
  _TCU03_/10 -> sigBadCalibration/1(sigBadCalibration)  "<sigBadCalibration>"
  _TCU03_/11 -> sigSupervisorFault/1(sigSupervisorFault)  "<sigSupervisorFault>"
  _TCU03_/12 -> sigCoil3DriverOpenShort/1(sigCoil3DriverOpenShort)  "<sigCoil3DriverOpenShort>"
  _TCU03_/13 -> sigCoil4DriverOpenShort/1(sigCoil4DriverOpenShort)  "<sigCoil4DriverOpenShort>"
  _TCU03_/14 -> sigHighPedalDisable/1(sigHighPedalDisable)  "<sigHighPedalDisable>"
  _TCU03_/15 -> sigBrakeWiperLow/1(sigBrakeWiperLow)  "<sigBrakeWiperLow>"
  _TCU03_/16 -> sigBrakeWiperHigh/1(sigBrakeWiperHigh)  "<sigBrakeWiperHigh>"
  _TCU03_/17 -> sigStallDetected/1(sigStallDetected)  "<sigStallDetected>"
  _TCU03_/18 -> sigParameterChangeFault/1(sigParameterChangeFault)  "<sigParameterChangeFault>"
  _TCU03_/19 -> sigMotorCharacterization/1(sigMotorCharacterization)  "<sigMotorCharacterization>"
  _TCU03_/20 -> sigVCLRunTimeError/1(sigVCLRunTimeError)  "<sigVCLRunTimeError>"
  _TCU03_/21 -> sigEEPROMFailure/1(sigEEPROMFailure)  "<sigEEPROMFailure>"
  _TCU03_/22 -> sigThrottlewiperLow/1(sigThrottlewiperLow)  "<sigThrottlewiperLow>"
  _TCU03_/23 -> sigThrottlewiperHigh/1(sigThrottlewiperHigh)  "<sigThrottlewiperHigh>"
  _TCU03_/24 -> sigMainContactordidnotClose/1(sigMainContactordidnotClose)  "<sigMainContactordidnotClose>"
  _TCU03_/25 -> sigMainContactorWelded/1(sigMainContactorWelded)  "<sigMainContactorWelded>"
  _TCU03_/26 -> sigMotorPhaseOpen/1(sigMotorPhaseOpen)  "<sigMotorPhaseOpen>"
  _TCU03_/27 -> sigSinCosSensorFault/1(sigSinCosSensorFault)  "<sigSinCosSensorFault>"
  _TCU03_/28 -> sigMainOpenShort/1(sigMainOpenShort)  "<sigMainOpenShort>"
  _TCU03_/29 -> sigMotorTempSensorFault/1(sigMotorTempSensorFault)  "<sigMotorTempSensorFault>"
  _TCU03_/30 -> sigMotorTempHotCutback/1(sigMotorTempHotCutback)  "<sigMotorTempHotCutback>"
  _TCU03_/31 -> sig5VSupplyFailure/1(sig5VSupplyFailure)  "<sig5VSupplyFailure>"
  _TCU03_/32 -> sigBPosOvervoltageCutback/1(sigBPosOvervoltageCutback)  "<sigBPosOvervoltageCutback>"
  _TCU03_/33 -> sigBPosUndervoltageCutback/1(sigBPosUndervoltageCutback)  "<sigBPosUndervoltageCutback>"
  _TCU03_/34 -> sigControllerOvertempCutback/1(sigControllerOvertempCutback)  "<sigControllerOvertempCutback>"
  _TCU03_/35 -> sigSevereKSIOvervoltage/1(sigSevereKSIOvervoltage)  "<sigSevereKSIOvervoltage>"
  _TCU03_/36 -> sigSevereBPosOvervoltage/1(sigSevereBPosOvervoltage)  "<sigSevereBPosOvervoltage>"
  _TCU03_/37 -> sigSevereKSIUndervoltage/1(sigSevereKSIUndervoltage)  "<sigSevereKSIUndervoltage>"
  _TCU03_/38 -> sigSevereBPosUndervoltage/1(sigSevereBPosUndervoltage)  "<sigSevereBPosUndervoltage>"
  _TCU03_/39 -> sigControllerSevereOvertemp/1(sigControllerSevereOvertemp)  "<sigControllerSevereOvertemp>"
  _TCU03_/40 -> sigControllerSevereUndertemp/1(sigControllerSevereUndertemp)  "<sigControllerSevereUndertemp>"
  _TCU03_/41 -> sigPrechargeFailed/1(sigPrechargeFailed)  "<sigPrechargeFailed>"
  _TCU03_/42 -> sigCurrentSensorFault/1(sigCurrentSensorFault)  "<sigCurrentSensorFault>"
  _TCU03_/43 -> sigControllerOverCurrent/1(sigControllerOverCurrent)  "<sigControllerOverCurrent>"
  _TCU03_/44 -> sigControllerCommonFault/1(sigControllerCommonFault)  "<sigControllerCommonFault>"

== system DriveSystemControl/Bus Configuration (1) - Out/Simulated ECUs/gitam Controller CAN File 08082024/Telematics/RX/PDUs/TCU04 ==
  TCU04 : Inport
  _TCU04_ : BusSelector  OutputSignals=sigMCU5_Efficiency,sigMCU5_Hillhold,sigMCU5_Speed,sigMCU5_RegenFlag,sigMCU5_DriveMode
  sigMCU5_DriveMode : Subsystem
  sigMCU5_Efficiency : Subsystem
  sigMCU5_Hillhold : Subsystem
  sigMCU5_RegenFlag : Subsystem
  sigMCU5_Speed : Subsystem
  wires:
  TCU04/1 -> _TCU04_/1  "TCU04"
  _TCU04_/1 -> sigMCU5_Efficiency/1(sigMCU5_Efficiency)  "<sigMCU5_Efficiency>"
  _TCU04_/2 -> sigMCU5_Hillhold/1(sigMCU5_Hillhold)  "<sigMCU5_Hillhold>"
  _TCU04_/3 -> sigMCU5_Speed/1(sigMCU5_Speed)  "<sigMCU5_Speed>"
  _TCU04_/4 -> sigMCU5_RegenFlag/1(sigMCU5_RegenFlag)  "<sigMCU5_RegenFlag>"
  _TCU04_/5 -> sigMCU5_DriveMode/1(sigMCU5_DriveMode)  "<sigMCU5_DriveMode>"

== system DriveSystemControl/Bus Configuration (1) - Out/Simulated ECUs/gitam Controller CAN File 08082024/Telematics/RX/PDUs/TCU05 ==
  TCU05 : Inport
  _TCU05_ : BusSelector  OutputSignals=sigMCU6_Odometer
  sigMCU6_Odometer : Subsystem
  wires:
  TCU05/1 -> _TCU05_/1  "TCU05"
  _TCU05_/1 -> sigMCU6_Odometer/1(sigMCU6_Odometer)  "<sigMCU6_Odometer>"

== system DriveSystemControl/Bus Configuration (1) - In/Manipulation/gitam Controller CAN File 08082024/WIP/CANChannel/PDUs/BMS01/sigBatteryMalfunctionLight ==
  Feature Switch : Subsystem
  ISignal Overwrite Value : Subsystem
  _sigBatteryMalfunctionLight_ : BusCreator  Inputs=2
  sigBatteryMalfunctionLight : Outport
  wires:
  _sigBatteryMalfunctionLight_/1 -> sigBatteryMalfunctionLight/1  "sigBatteryMalfunctionLight"
  Feature Switch/1(Feature Switch) -> _sigBatteryMalfunctionLight_/1  "Feature Switch"
  ISignal Overwrite Value/1(ISignal Overwrite Value) -> _sigBatteryMalfunctionLight_/2  "ISignal Overwrite Value"

== system DriveSystemControl/Bus Configuration (1) - In/Manipulation/gitam Controller CAN File 08082024/WIP/CANChannel/PDUs/BMS01/sigKeyOnIndicator ==
  Feature Switch : Subsystem
  ISignal Overwrite Value : Subsystem
  _sigKeyOnIndicator_ : BusCreator  Inputs=2
  sigKeyOnIndicator : Outport
  wires:
  _sigKeyOnIndicator_/1 -> sigKeyOnIndicator/1  "sigKeyOnIndicator"
  Feature Switch/1(Feature Switch) -> _sigKeyOnIndicator_/1  "Feature Switch"
  ISignal Overwrite Value/1(ISignal Overwrite Value) -> _sigKeyOnIndicator_/2  "ISignal Overwrite Value"

== system DriveSystemControl/Bus Configuration (1) - In/Manipulation/gitam Controller CAN File 08082024/WIP/CANChannel/PDUs/BMS01/sigStateOfCharge ==
  Feature Switch : Subsystem
  ISignal Overwrite Value : Subsystem
  _sigStateOfCharge_ : BusCreator  Inputs=2
  sigStateOfCharge : Outport
  wires:
  _sigStateOfCharge_/1 -> sigStateOfCharge/1  "sigStateOfCharge"
  Feature Switch/1(Feature Switch) -> _sigStateOfCharge_/1  "Feature Switch"
  ISignal Overwrite Value/1(ISignal Overwrite Value) -> _sigStateOfCharge_/2  "ISignal Overwrite Value"

== system DriveSystemControl/Bus Configuration (1) - In/Manipulation/gitam Controller CAN File 08082024/WIP/CANChannel/PDUs/BMS02/sigBatteryCurrent ==
  Feature Switch : Subsystem
  ISignal Overwrite Value : Subsystem
  _sigBatteryCurrent_ : BusCreator  Inputs=2
  sigBatteryCurrent : Outport
  wires:
  _sigBatteryCurrent_/1 -> sigBatteryCurrent/1  "sigBatteryCurrent"
  Feature Switch/1(Feature Switch) -> _sigBatteryCurrent_/1  "Feature Switch"
  ISignal Overwrite Value/1(ISignal Overwrite Value) -> _sigBatteryCurrent_/2  "ISignal Overwrite Value"

== system DriveSystemControl/Bus Configuration (1) - In/Manipulation/gitam Controller CAN File 08082024/WIP/CANChannel/PDUs/BMS02/sigDriveCurrentLimit ==
  Feature Switch : Subsystem
  ISignal Overwrite Value : Subsystem
  _sigDriveCurrentLimit_ : BusCreator  Inputs=2
  sigDriveCurrentLimit : Outport
  wires:
  _sigDriveCurrentLimit_/1 -> sigDriveCurrentLimit/1  "sigDriveCurrentLimit"
  Feature Switch/1(Feature Switch) -> _sigDriveCurrentLimit_/1  "Feature Switch"
  ISignal Overwrite Value/1(ISignal Overwrite Value) -> _sigDriveCurrentLimit_/2  "ISignal Overwrite Value"

== system DriveSystemControl/Bus Configuration (1) - In/Manipulation/gitam Controller CAN File 08082024/WIP/CANChannel/PDUs/BMS02/sigRegenCurrentLimit ==
  Feature Switch : Subsystem
  ISignal Overwrite Value : Subsystem
  _sigRegenCurrentLimit_ : BusCreator  Inputs=2
  sigRegenCurrentLimit : Outport
  wires:
  _sigRegenCurrentLimit_/1 -> sigRegenCurrentLimit/1  "sigRegenCurrentLimit"
  Feature Switch/1(Feature Switch) -> _sigRegenCurrentLimit_/1  "Feature Switch"
  ISignal Overwrite Value/1(ISignal Overwrite Value) -> _sigRegenCurrentLimit_/2  "ISignal Overwrite Value"

== system DriveSystemControl/Bus Configuration (1) - In/Manipulation/gitam Controller CAN File 08082024/WIP/CANChannel/PDUs/BMS02/sigVehicleModeRequest ==
  Feature Switch : Subsystem
  ISignal Overwrite Value : Subsystem
  _sigVehicleModeRequest_ : BusCreator  Inputs=2
  sigVehicleModeRequest : Outport
  wires:
  _sigVehicleModeRequest_/1 -> sigVehicleModeRequest/1  "sigVehicleModeRequest"
  Feature Switch/1(Feature Switch) -> _sigVehicleModeRequest_/1  "Feature Switch"
  ISignal Overwrite Value/1(ISignal Overwrite Value) -> _sigVehicleModeRequest_/2  "ISignal Overwrite Value"

== system DriveSystemControl/Bus Configuration (1) - In/Manipulation/gitam Controller CAN File 08082024/WIP/CANChannel/PDUs/MainController/CCU_heartBeat ==
  Feature Switch : Subsystem
  ISignal Overwrite Value : Subsystem
  _CCU_heartBeat_ : BusCreator  Inputs=2
  CCU_heartBeat : Outport
  wires:
  _CCU_heartBeat_/1 -> CCU_heartBeat/1  "CCU_heartBeat"
  Feature Switch/1(Feature Switch) -> _CCU_heartBeat_/1  "Feature Switch"
  ISignal Overwrite Value/1(ISignal Overwrite Value) -> _CCU_heartBeat_/2  "ISignal Overwrite Value"
